simulink model "Validation_de_modele"  (R2023b)
settings: Solver=VariableStepAuto  StartTime=0.0  StopTime=0.5  RelTol=1e-3
InitFcn:
  | C=4000e-6;
  | L=40e-3;
  | R=10;
  | E=12;
  | f=1e3;
libraries: spsSeriesRLCBranchLib x3, spsVoltageMeasurementLib x2, spsDCVoltageSourceLib x1, spsDiodeLib x1, spsGroundLib x1, spsIdealSwitchLib x1, eePwmGenerator x1, spsCurrentMeasurementLib x1, sps_lib x1
settings Model: Creator=lenovo  LastModifiedBy=lenovo

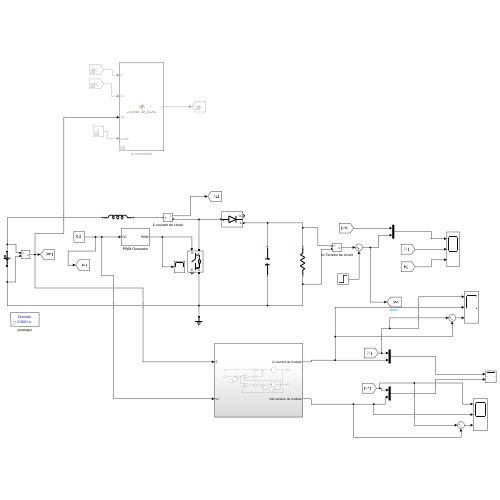
[thumbnail: Simulink's stored preview of the top-level diagram]
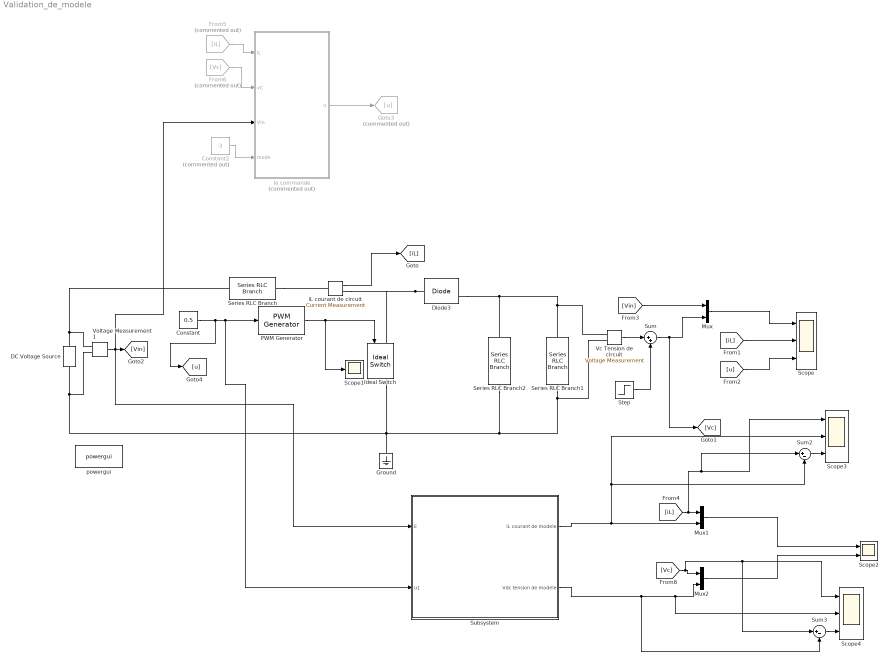
== system Validation_de_modele ==
  Constant : Constant  Value=0.5
  Constant2 : Constant  Commented=on  Value=3
  DC Voltage Source : spsDCVoltageSourceLib/DC Voltage Source  Amplitude=E  Measurements=None
  Diode3 : spsDiodeLib/Diode  Ron=1e-6  Lon=0  Vf=0  IC=0  UseSnubber=0  Rs=0  Cs=0  Measurements=on
  From5 : From  Commented=on  GotoTag=iL
  From6 : From  Commented=on  GotoTag=Vc
  Goto3 : Goto  Commented=on  GotoTag=u
  Ground : spsGroundLib/Ground  LConnTagsString=a
  Ideal Switch : spsIdealSwitchLib/Ideal Switch  Ron=0.001  Lon=0  IC=0  Rs=1e5  Cs=inf  Measurements=on
  Mux : Mux  Inputs=2
  Mux1 : Mux  Inputs=2
  Mux2 : Mux  Inputs=2
  PWM Generator : eePwmGenerator/PWM Generator  CarrCount=Up  Tper=1/f  Tdelay=0  Ts=1e-7
  Scope : Scope  NumInputPorts=3
  Scope1 : Scope
  Scope2 : Scope  NumInputPorts=2
  Scope3 : Scope  NumInputPorts=3
  Scope4 : Scope  NumInputPorts=3
  Series RLC Branch : spsSeriesRLCBranchLib/Series RLC Branch  LConnTagsString=__new0  RConnTagsString=__new0  BranchType=L  Resistance=1  Inductance=L  SetiL0=off  InitialCurrent=0  Capacitance=1e-6  Setx0=off  InitialVoltage=0  Measurements=None
  Series RLC Branch1 : spsSeriesRLCBranchLib/Series RLC Branch  LConnTagsString=__new0  RConnTagsString=__new0  BranchType=R  Resistance=R  Inductance=1e-3  SetiL0=off  InitialCurrent=0  Capacitance=1e-6  Setx0=off  InitialVoltage=0  Measurements=None
  Series RLC Branch2 : spsSeriesRLCBranchLib/Series RLC Branch  LConnTagsString=__new0  RConnTagsString=__new0  BranchType=C  Resistance=1  Inductance=1e-3  SetiL0=off  InitialCurrent=0  Capacitance=C  Setx0=off  InitialVoltage=0  Measurements=None
  Step : Step  Time=0.01  After=0  SampleTime=0
  Subsystem : Subsystem
  Sum : Sum  Inputs=|++
  Sum2 : Sum  Inputs=|+-
  Sum3 : Sum  Inputs=|+-
  Vc Tension de circuit : spsVoltageMeasurementLib/Voltage Measurement  PhasorSimulation=off  OutputType=Complex  PSBequivalent=0
  Voltage Measurement1 : spsVoltageMeasurementLib/Voltage Measurement  PhasorSimulation=off  OutputType=Complex  PSBequivalent=0
  iL courant de circuit : spsCurrentMeasurementLib/Current Measurement  PhasorSimulation=off  OutputType=Complex  PSBequivalent=0
  la commande : MATLAB Function  Commented=on  TreatAsAtomicUnit=on
  powergui : sps_lib/powergui  Priority=1  SimulationMode=Discrete  SampleTime=1e-4  frequency=60  Iterations=50  frequencyindice=0  Pbase=100e6  ErrMax=1e-4  UnitsV=kV  UnitsW=MW  buscounter=0  FunctionMessages=off  echomessages=off  EnableUseOfTLC=off  CurrentSourceSwitches=off  DisableSnubberDevices=off  DisableRonSwitches=off  DisableVfSwitches=off  DisplayEquations=off  AutomaticDiscreteSolvers=off  SolverType=Tustin/Backward Euler (TBE)  Interpol=off  ExternalGateDelay=off  methode=off  Ts=100  x0status=blocks  SPID=on  SwTol=0  HookPort=off  NonlinearTolerance=1e-4  nMaxIteration=100  ContinueOnMaxIteration=off  RestoreLinks=warning  ResistiveCurrentMeasurement=off  Frange=[0:2:500]  Ylog=off  Xlog=on  ShowGrid=off  save=off  variable=ZData  structure=0  ZoomFFT=off  StartTime=0.0  cycles=1  DisplayStyle=1  fundamental=60  FreqAxis=off  MaxFrequency=1000  frequencyindicesteady=1  RmsSteady=1  display=off
  wires:
  PWM Generator/1 -> Scope1/1, Ideal Switch/1
  [Vin] -> Mux/1
  Vc Tension de circuit/1 -> Sum/1
  iL courant de circuit/1 -> [iL]
  [iL] -> Scope/2
  Mux/1 -> Scope/1
  [u] -> Scope/3
  Subsystem/1(iL courant de modele) -> Sum2/2, Scope3/2, Mux1/2
  Mux1/1 -> Scope2/1
  Mux2/1 -> Scope2/2
  [iL] -> Sum2/1, Scope3/1, Mux1/1
  Sum/1 -> [Vc], Mux/2
  Step/1 -> Sum/2
  Sum2/1 -> Scope3/3
  [Vc] -> Sum3/1, Scope4/1, Mux2/1
  Subsystem/2(Vdc tension de modele) -> Sum3/2, Scope4/2, Mux2/2
  Sum3/1 -> Scope4/3
  Constant2/1 -> la commande/4(mode)
  From6/1 -> la commande/2(vC)
  Voltage Measurement1/1 -> la commande/3(Vin), Subsystem/1(E), [Vin]
  From5/1 -> la commande/1(iL)
  la commande/1(u) -> Goto3/1
  Constant/1 -> [u], Subsystem/2(u1), PWM Generator/1
  connections:
  Series RLC Branch/LConn1 -- Voltage Measurement1/LConn1 -- DC Voltage Source/RConn1
  Diode3/LConn1 -- iL courant de circuit/RConn1 -- Ideal Switch/LConn1
  Diode3/RConn1 -- Series RLC Branch2/LConn1 -- Vc Tension de circuit/LConn1 -- Series RLC Branch1/LConn1
  Series RLC Branch1/RConn1 -- Vc Tension de circuit/LConn2 -- Series RLC Branch2/RConn1 -- Ground/LConn1 -- Ideal Switch/RConn1 -- Voltage Measurement1/LConn2 -- DC Voltage Source/LConn1
  Series RLC Branch/RConn1 -- iL courant de circuit/LConn1

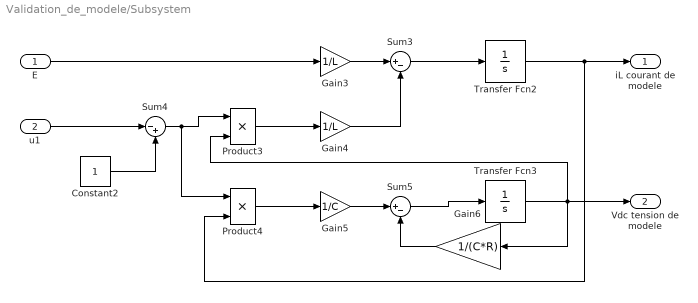
== system Validation_de_modele/Subsystem ==
  E : Inport
  u1 : Inport  Port=2
  Constant2 : Constant
  Gain3 : Gain  Gain=1/L
  Gain4 : Gain  Gain=1/L
  Gain5 : Gain  Gain=1/C
  Gain6 : Gain  Gain=1/(C*R)
  Product3 : Product
  Product4 : Product
  Sum3 : Sum  Inputs=|+-
  Sum4 : Sum  Inputs=|-+
  Sum5 : Sum  Inputs=|+-
  Transfer Fcn2 : TransferFcn  Denominator=[1 0]
  Transfer Fcn3 : TransferFcn  Denominator=[1 0]
  iL courant de modele : Outport
  Vdc tension de modele : Outport  Port=2
  wires:
  E/1 -> Gain3/1
  Gain3/1 -> Sum3/1
  Gain4/1 -> Sum3/2
  u1/1 -> Sum4/1
  Constant2/1 -> Sum4/2
  Product3/1 -> Gain4/1
  Sum4/1 -> Product4/1, Product3/1
  Product4/1 -> Gain5/1
  Gain5/1 -> Sum5/1
  Gain6/1 -> Sum5/2
  Sum3/1 -> Transfer Fcn2/1
  Transfer Fcn2/1 -> Product4/2, iL courant de modele/1
  Sum5/1 -> Transfer Fcn3/1
  Transfer Fcn3/1 -> Product3/2, Gain6/1, Vdc tension de modele/1

== matlab function Validation_de_modele/la commande ==
  data: iL input; u output; vC input; Vin input; mode input
function u = commande_boost(iL, vC, Vin, mode)
% COMMANDE_BOOST
% Loi de commande non linéaire pour un convertisseur Boost.
%
% Entrées :
%   iL   : courant dans l'inductance (A)
%   vC   : tension de sortie (V)
%   Vin  : tension d'entrée instantanée (V)
%   mode : sélection de la loi de commande
%       1: commande à l'équilibre (u = u_eq)
%       2: Lyapunov : annulation complète de Vdot
%       3: Lyapunov : annulation des termes non stabilisants
%
% Sortie :
% u    : rapport cyclique


%% Paramètres de fonctionnement
R    = 10;    % résistance de charge (ohms)
Vref = 24;    % tension de sortie désirée (V)

%% 1) Point d'équilibre associé à Vref
u_eq  = 1 - Vin./Vref;      % duty à l'équilibre
iL_eq = Vref.^2./(R*Vin);   % courant inductif à l'équilibre
vC_eq = Vref;               % tension de sortie à l'équilibre

%% 2) Changement de Variables 
tilde_iL = iL - iL_eq;
tilde_vC = vC - vC_eq;

% Le terme non stable
w = vC_eq*tilde_iL - iL_eq*tilde_vC;

%% 3) Paramètres des lois de commande
alpha1 = 50;    % gain Lyapunov (commande 2) sur tilde_iL^2
alpha2 = 1.0;   % gain Lyapunov (commande 2) sur tilde_vC^2
k      = 0.5;   % gain Lyapunov (commande 3) sur w

%% 4) Sélection de la loi de commande
switch mode
    
    case 1
        % Mode 1 : duty simplement fixé à la valeur d'équilibre
        u = u_eq;
        
    case 2
        % Mode 2 : annulation complète de Vdot
        
        num = -alpha1*tilde_iL.^2 - (alpha2 - 1/R).*tilde_vC.^2;
        
        if abs(w) < 1e-6
            % si le dénominateur est trop petit, on évite la division
            u = u_eq;
        else
            u = u_eq + num./w;
        end
       
    case 3
        % Mode 3 : annulation des seuls termes non stabilisants
     
        u = u_eq - k*w;
        
    otherwise
        % mode non reconnu : on se rabat sur la commande à l'équilibre
        u = u_eq;
end

%% 5) Saturation du duty dans l'intervalle physique
u = max(min(u, 0.95), 0.05);

end
